simulink model "WSCC_Indian_400kV_Legacy"  (R2022a)
settings: Solver=FixedStepDiscrete  StartTime=0.0  StopTime=1  FixedStep=5e-7  RelTol=1e-3
PreLoadFcn:
  | tf=1e-3
  | to=20e-3
model workspace (MAT data in the model file):
  tf = 0.001
  to = 0.02
undefined symbols (not defined in the file or in its folder): D1, Delta
libraries: spsFourierLib x72, spsPowerPositiveSequenceLib x24, spsThreePhaseVIMeasurementLib x21, spsThreePhaseBreakerLib x12, spsDistributedParametersLineLib x12, spsLoadFlowBusLib x9, spsRMSLib x6, spsThreePhaseParallelRLCLoadLib x6, spsThreePhaseSeriesRLCLoadLib x3, spsThreePhaseSourceLib x3, spsThreePhaseTransformerTwoWindingsLib x3, spsThreePhaseFaultLib x1
(part 2 of 2)

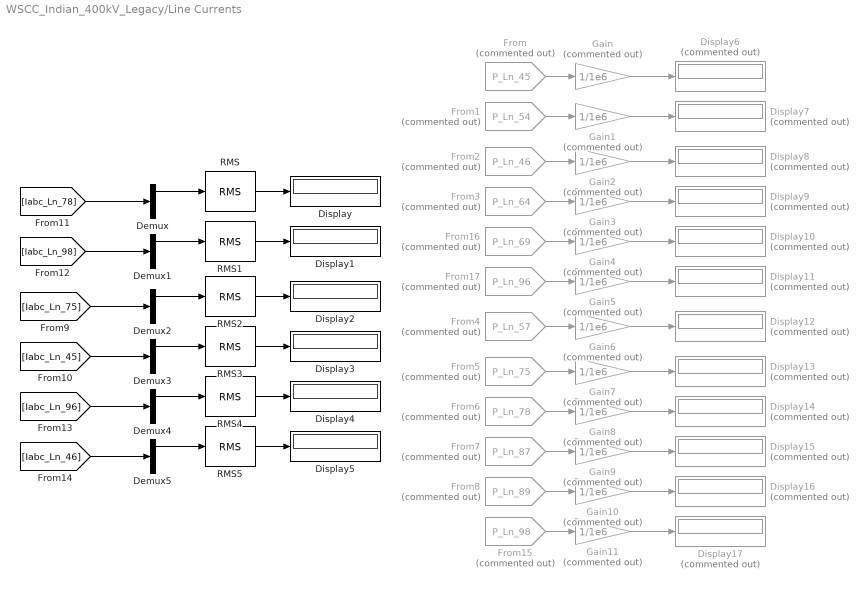
== system WSCC_Indian_400kV_Legacy/Line Currents ==
  Demux{,1..5} (6 alike) : Demux  Outputs=3
  Display{,1..5} (6 alike) : Display
  Display{6..17} (12 alike) : Display  Commented=on
  From : From  Commented=on  GotoTag=P_Ln_45  TagVisibility=global
  From1 : From  Commented=on  GotoTag=P_Ln_54  TagVisibility=global
  From15 : From  Commented=on  GotoTag=P_Ln_98  TagVisibility=global
  From16 : From  Commented=on  GotoTag=P_Ln_69  TagVisibility=global
  From17 : From  Commented=on  GotoTag=P_Ln_96  TagVisibility=global
  From2 : From  Commented=on  GotoTag=P_Ln_46  TagVisibility=global
  From3 : From  Commented=on  GotoTag=P_Ln_64  TagVisibility=global
  From4 : From  Commented=on  GotoTag=P_Ln_57  TagVisibility=global
  From5 : From  Commented=on  GotoTag=P_Ln_75  TagVisibility=global
  From6 : From  Commented=on  GotoTag=P_Ln_78  TagVisibility=global
  From7 : From  Commented=on  GotoTag=P_Ln_87  TagVisibility=global
  From8 : From  Commented=on  GotoTag=P_Ln_89  TagVisibility=global
  Gain{,1..11} (12 alike) : Gain  Commented=on  Gain=1/1e6
  RMS{,1..5} (6 alike) : spsRMSLib/RMS  TrueRMS=off  Freq=50  RMSInit=120  Ts=0
  wires:
  [Iabc_Ln_96] -> Demux4/1
  RMS4/1 -> Display4/1
  Demux5/1 -> RMS5/1
  Demux2/1 -> RMS2/1
  [Iabc_Ln_78] -> Demux/1
  Demux4/1 -> RMS4/1
  Demux3/1 -> RMS3/1
  RMS2/1 -> Display2/1
  RMS3/1 -> Display3/1
  Demux1/1 -> RMS1/1
  RMS1/1 -> Display1/1
  Demux/1 -> RMS/1
  [Iabc_Ln_46] -> Demux5/1
  [Iabc_Ln_45] -> Demux3/1
  [Iabc_Ln_75] -> Demux2/1
  [Iabc_Ln_98] -> Demux1/1
  RMS/1 -> Display/1
  RMS5/1 -> Display5/1
  From/1 -> Gain/1
  From1/1 -> Gain1/1
  From2/1 -> Gain2/1
  From3/1 -> Gain3/1
  From16/1 -> Gain4/1
  From17/1 -> Gain5/1
  From4/1 -> Gain6/1
  From5/1 -> Gain7/1
  From6/1 -> Gain8/1
  From7/1 -> Gain9/1
  From8/1 -> Gain10/1
  From15/1 -> Gain11/1
  Gain/1 -> Display6/1
  Gain1/1 -> Display7/1
  Gain2/1 -> Display8/1
  Gain3/1 -> Display9/1
  Gain4/1 -> Display10/1
  Gain5/1 -> Display11/1
  Gain6/1 -> Display12/1
  Gain7/1 -> Display13/1
  Gain8/1 -> Display14/1
  Gain9/1 -> Display15/1
  Gain10/1 -> Display16/1
  Gain11/1 -> Display17/1

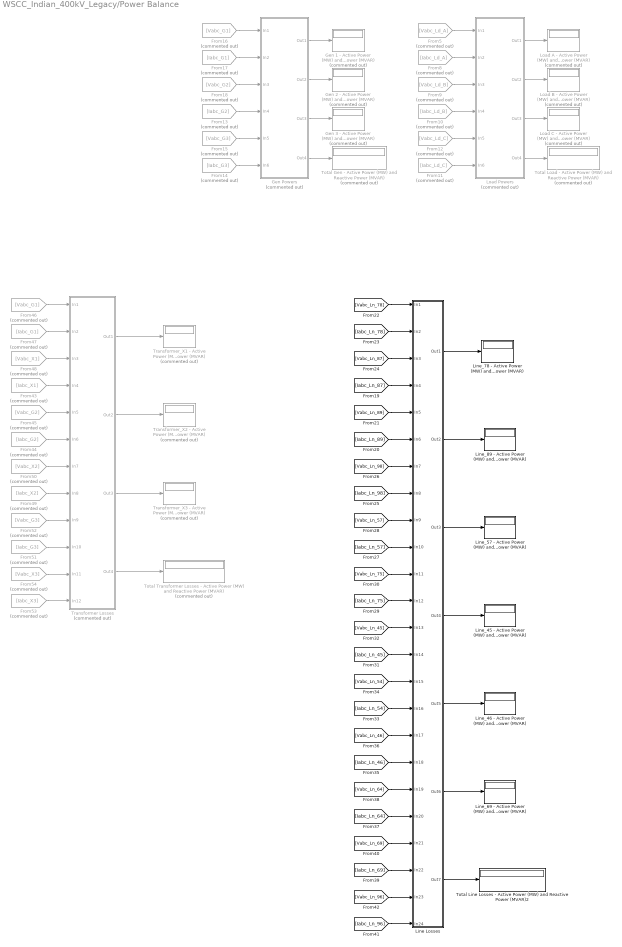
== system WSCC_Indian_400kV_Legacy/Power Balance ==
  From10 : From  Commented=on  GotoTag=Iabc_Ld_B  TagVisibility=global
  From11 : From  Commented=on  GotoTag=Iabc_Ld_C  TagVisibility=global
  From12 : From  Commented=on  GotoTag=Vabc_Ld_C  TagVisibility=global
  From13 : From  Commented=on  GotoTag=Iabc_G2  TagVisibility=global
  From14 : From  Commented=on  GotoTag=Iabc_G3  TagVisibility=global
  From15 : From  Commented=on  GotoTag=Vabc_G3  TagVisibility=global
  From16 : From  Commented=on  GotoTag=Vabc_G1  TagVisibility=global
  From17 : From  Commented=on  GotoTag=Iabc_G1  TagVisibility=global
  From18 : From  Commented=on  GotoTag=Vabc_G2  TagVisibility=global
  From43 : From  Commented=on  GotoTag=Iabc_X1  TagVisibility=global
  From44 : From  Commented=on  GotoTag=Iabc_G2  TagVisibility=global
  From45 : From  Commented=on  GotoTag=Vabc_G2  TagVisibility=global
  From46 : From  Commented=on  GotoTag=Vabc_G1  TagVisibility=global
  From47 : From  Commented=on  GotoTag=Iabc_G1  TagVisibility=global
  From48 : From  Commented=on  GotoTag=Vabc_X1  TagVisibility=global
  From49 : From  Commented=on  GotoTag=Iabc_X2  TagVisibility=global
  From5 : From  Commented=on  GotoTag=Vabc_Ld_A  TagVisibility=global
  From50 : From  Commented=on  GotoTag=Vabc_X2  TagVisibility=global
  From51 : From  Commented=on  GotoTag=Iabc_G3  TagVisibility=global
  From52 : From  Commented=on  GotoTag=Vabc_G3  TagVisibility=global
  From53 : From  Commented=on  GotoTag=Iabc_X3  TagVisibility=global
  From54 : From  Commented=on  GotoTag=Vabc_X3  TagVisibility=global
  From8 : From  Commented=on  GotoTag=Iabc_Ld_A  TagVisibility=global
  From9 : From  Commented=on  GotoTag=Vabc_Ld_B  TagVisibility=global
  Gen 1 - Active Power (MW) and Reactive Power (MVAR) : Display  Commented=on
  Gen 2 - Active Power (MW) and Reactive Power (MVAR) : Display  Commented=on
  Gen 3 - Active Power (MW) and Reactive Power (MVAR) : Display  Commented=on
  Gen Powers : Subsystem  Commented=on
  Line Losses : Subsystem
  Line_45 - Active Power (MW) and Reactive Power (MVAR) : Display
  Line_46 - Active Power (MW) and Reactive Power (MVAR) : Display
  Line_57 - Active Power (MW) and Reactive Power (MVAR) : Display
  Line_69 - Active Power (MW) and Reactive Power (MVAR) : Display
  Line_78 - Active Power (MW) and Reactive Power (MVAR) : Display
  Line_89 - Active Power (MW) and Reactive Power (MVAR) : Display
  Load A - Active Power (MW) and Reactive Power (MVAR) : Display  Commented=on
  Load B - Active Power (MW) and Reactive Power (MVAR) : Display  Commented=on
  Load C - Active Power (MW) and Reactive Power (MVAR) : Display  Commented=on
  Load Powers : Subsystem  Commented=on
  Total Gen - Active Power (MW) and Reactive Power (MVAR) : Display  Commented=on
  Total Line Losses - Active Power (MW) and Reactive Power (MVAR)2 : Display
  Total Load - Active Power (MW) and Reactive Power (MVAR) : Display  Commented=on
  Total Transformer Losses - Active Power (MW) and Reactive Power (MVAR) : Display  Commented=on
  Transformer Losses : Subsystem  Commented=on
  Transformer_X1 - Active Power (MW) and Reactive Power (MVAR) : Display  Commented=on
  Transformer_X2 - Active Power (MW) and Reactive Power (MVAR) : Display  Commented=on
  Transformer_X3 - Active Power (MW) and Reactive Power (MVAR) : Display  Commented=on
  wires:
  From44/1 -> Transformer Losses/6(In6)
  [Iabc_Ln_45] -> Line Losses/14(In14)
  From16/1 -> Gen Powers/1(In1)
  [Iabc_Ln_75] -> Line Losses/12(In12)
  Transformer Losses/1(Out1) -> Transformer_X1 - Active Power (MW) and Reactive Power (MVAR)/1
  Transformer Losses/4(Out4) -> Total Transformer Losses - Active Power (MW) and Reactive Power (MVAR)/1
  [Iabc_Ln_54] -> Line Losses/16(In16)
  [Vabc_Ln_54] -> Line Losses/15(In15)
  [Vabc_Ln_87] -> Line Losses/3(In3)
  From10/1 -> Load Powers/4(In4)
  [Vabc_Ln_98] -> Line Losses/7(In7)
  From11/1 -> Load Powers/6(In6)
  Line Losses/4(Out4) -> Line_45 - Active Power (MW) and Reactive Power (MVAR)/1
  Load Powers/4(Out4) -> Total Load - Active Power (MW) and Reactive Power (MVAR)/1
  Load Powers/3(Out3) -> Load C - Active Power (MW) and Reactive Power (MVAR)/1
  [Vabc_Ln_64] -> Line Losses/19(In19)
  From50/1 -> Transformer Losses/7(In7)
  Transformer Losses/2(Out2) -> Transformer_X2 - Active Power (MW) and Reactive Power (MVAR)/1
  [Vabc_Ln_57] -> Line Losses/9(In9)
  Line Losses/7(Out7) -> Total Line Losses - Active Power (MW) and Reactive Power (MVAR)2/1
  From48/1 -> Transformer Losses/3(In3)
  Load Powers/1(Out1) -> Load A - Active Power (MW) and Reactive Power (MVAR)/1
  From9/1 -> Load Powers/3(In3)
  [Iabc_Ln_46] -> Line Losses/18(In18)
  [Iabc_Ln_57] -> Line Losses/10(In10)
  [Iabc_Ln_69] -> Line Losses/22(In22)
  From52/1 -> Transformer Losses/9(In9)
  [Iabc_Ln_89] -> Line Losses/6(In6)
  Line Losses/2(Out2) -> Line_89 - Active Power (MW) and Reactive Power (MVAR)/1
  [Iabc_Ln_87] -> Line Losses/4(In4)
  From15/1 -> Gen Powers/5(In5)
  From18/1 -> Gen Powers/3(In3)
  [Vabc_Ln_69] -> Line Losses/21(In21)
  From51/1 -> Transformer Losses/10(In10)
  Transformer Losses/3(Out3) -> Transformer_X3 - Active Power (MW) and Reactive Power (MVAR)/1
  [Vabc_Ln_46] -> Line Losses/17(In17)
  Gen Powers/4(Out4) -> Total Gen - Active Power (MW) and Reactive Power (MVAR)/1
  [Iabc_Ln_98] -> Line Losses/8(In8)
  [Vabc_Ln_78] -> Line Losses/1(In1)
  From47/1 -> Transformer Losses/2(In2)
  From13/1 -> Gen Powers/4(In4)
  From53/1 -> Transformer Losses/12(In12)
  [Vabc_Ln_45] -> Line Losses/13(In13)
  From54/1 -> Transformer Losses/11(In11)
  [Iabc_Ln_96] -> Line Losses/24(In24)
  [Vabc_Ln_96] -> Line Losses/23(In23)
  From49/1 -> Transformer Losses/8(In8)
  [Vabc_Ln_75] -> Line Losses/11(In11)
  Gen Powers/1(Out1) -> Gen 1 - Active Power (MW) and Reactive Power (MVAR)/1
  [Vabc_Ln_89] -> Line Losses/5(In5)
  From8/1 -> Load Powers/2(In2)
  [Iabc_Ln_64] -> Line Losses/20(In20)
  From46/1 -> Transformer Losses/1(In1)
  From17/1 -> Gen Powers/2(In2)
  Line Losses/1(Out1) -> Line_78 - Active Power (MW) and Reactive Power (MVAR)/1
  Line Losses/3(Out3) -> Line_57 - Active Power (MW) and Reactive Power (MVAR)/1
  From45/1 -> Transformer Losses/5(In5)
  Line Losses/6(Out6) -> Line_69 - Active Power (MW) and Reactive Power (MVAR)/1
  [Iabc_Ln_78] -> Line Losses/2(In2)
  From14/1 -> Gen Powers/6(In6)
  Line Losses/5(Out5) -> Line_46 - Active Power (MW) and Reactive Power (MVAR)/1
  From43/1 -> Transformer Losses/4(In4)
  Gen Powers/3(Out3) -> Gen 3 - Active Power (MW) and Reactive Power (MVAR)/1
  Gen Powers/2(Out2) -> Gen 2 - Active Power (MW) and Reactive Power (MVAR)/1
  From5/1 -> Load Powers/1(In1)
  From12/1 -> Load Powers/5(In5)
  Load Powers/2(Out2) -> Load B - Active Power (MW) and Reactive Power (MVAR)/1

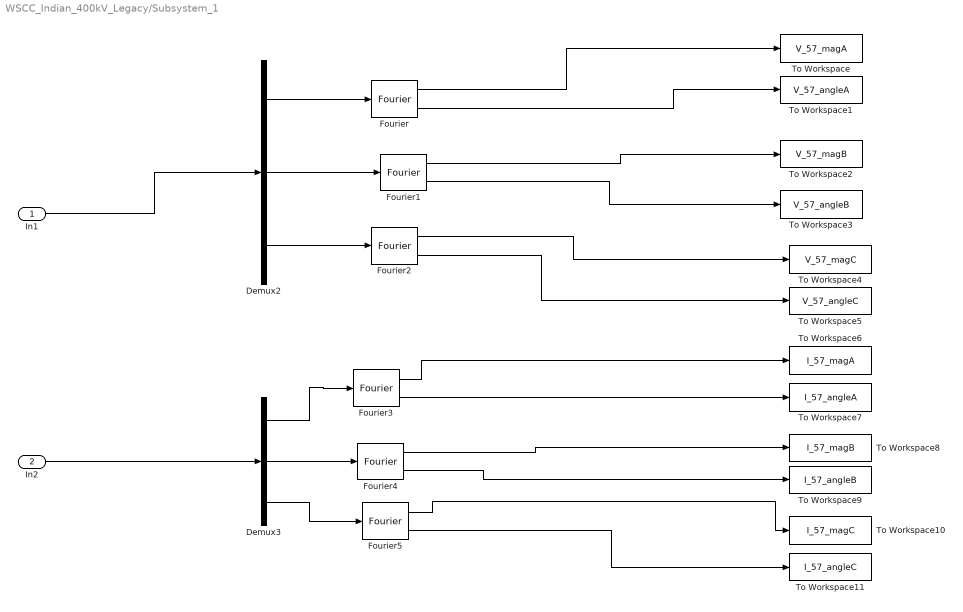
== system WSCC_Indian_400kV_Legacy/Subsystem_1 ==
  In1 : Inport
  In2 : Inport  Port=2
  Demux2 : Demux  Outputs=3
  Demux3 : Demux  Outputs=3
  Fourier{,1..5} (6 alike) : spsFourierLib/Fourier  Freq=50  n=1  InInit=[0, 0]  Ts=tf
      settings: SourceProductBaseCode=PS
  To Workspace : ToWorkspace  VariableName=V_57_magA  SaveFormat=Timeseries  SampleTime=to
  To Workspace1 : ToWorkspace  VariableName=V_57_angleA  SaveFormat=Timeseries  SampleTime=to
  To Workspace10 : ToWorkspace  VariableName=I_57_magC  SaveFormat=Timeseries  SampleTime=to
  To Workspace11 : ToWorkspace  VariableName=I_57_angleC  SaveFormat=Timeseries  SampleTime=to
  To Workspace2 : ToWorkspace  VariableName=V_57_magB  SaveFormat=Timeseries  SampleTime=to
  To Workspace3 : ToWorkspace  VariableName=V_57_angleB  SaveFormat=Timeseries  SampleTime=to
  To Workspace4 : ToWorkspace  VariableName=V_57_magC  SaveFormat=Timeseries  SampleTime=to
  To Workspace5 : ToWorkspace  VariableName=V_57_angleC  SaveFormat=Timeseries  SampleTime=to
  To Workspace6 : ToWorkspace  VariableName=I_57_magA  SaveFormat=Timeseries  SampleTime=to
  To Workspace7 : ToWorkspace  VariableName=I_57_angleA  SaveFormat=Timeseries  SampleTime=to
  To Workspace8 : ToWorkspace  VariableName=I_57_magB  SaveFormat=Timeseries  SampleTime=to
  To Workspace9 : ToWorkspace  VariableName=I_57_angleB  SaveFormat=Timeseries  SampleTime=to
  wires:
  Demux3/3 -> Fourier5/1
  Fourier4/1 -> To Workspace8/1
  Demux3/2 -> Fourier4/1
  Fourier3/2 -> To Workspace7/1
  Fourier5/1 -> To Workspace10/1
  Fourier3/1 -> To Workspace6/1
  Fourier5/2 -> To Workspace11/1
  Fourier4/2 -> To Workspace9/1
  Fourier2/2 -> To Workspace5/1
  Demux3/1 -> Fourier3/1
  Fourier2/1 -> To Workspace4/1
  Fourier1/2 -> To Workspace3/1
  Demux2/2 -> Fourier1/1
  Fourier/2 -> To Workspace1/1
  Fourier1/1 -> To Workspace2/1
  Demux2/3 -> Fourier2/1
  Fourier/1 -> To Workspace/1
  Demux2/1 -> Fourier/1
  In1/1 -> Demux2/1
  In2/1 -> Demux3/1

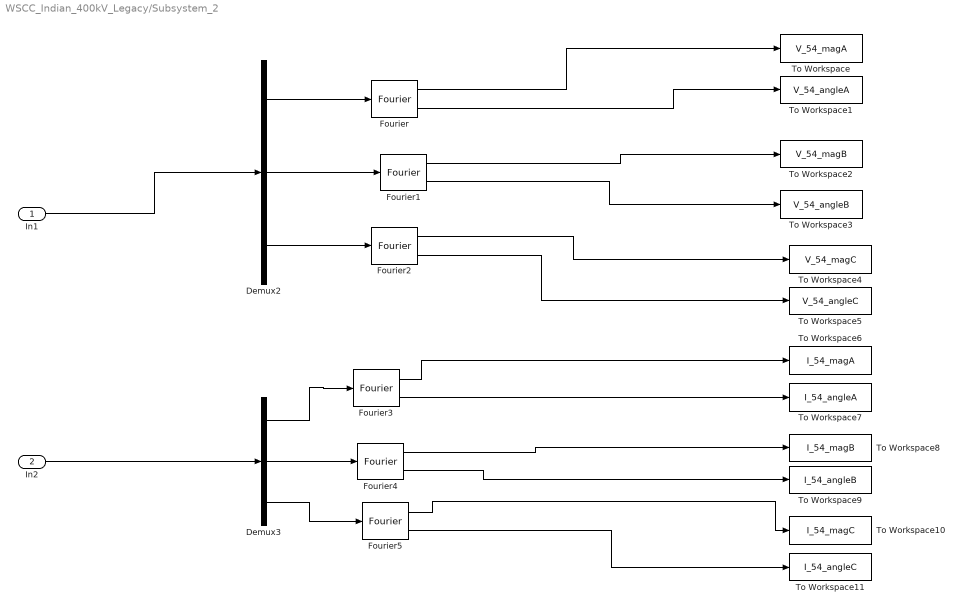
== system WSCC_Indian_400kV_Legacy/Subsystem_2 ==
  In1 : Inport
  In2 : Inport  Port=2
  Demux2 : Demux  Outputs=3
  Demux3 : Demux  Outputs=3
  Fourier{,1..5} (6 alike) : spsFourierLib/Fourier  Freq=50  n=1  InInit=[0, 0]  Ts=tf
      settings: SourceProductBaseCode=PS
  To Workspace : ToWorkspace  VariableName=V_54_magA  SaveFormat=Timeseries  SampleTime=to
  To Workspace1 : ToWorkspace  VariableName=V_54_angleA  SaveFormat=Timeseries  SampleTime=to
  To Workspace10 : ToWorkspace  VariableName=I_54_magC  SaveFormat=Timeseries  SampleTime=to
  To Workspace11 : ToWorkspace  VariableName=I_54_angleC  SaveFormat=Timeseries  SampleTime=to
  To Workspace2 : ToWorkspace  VariableName=V_54_magB  SaveFormat=Timeseries  SampleTime=to
  To Workspace3 : ToWorkspace  VariableName=V_54_angleB  SaveFormat=Timeseries  SampleTime=to
  To Workspace4 : ToWorkspace  VariableName=V_54_magC  SaveFormat=Timeseries  SampleTime=to
  To Workspace5 : ToWorkspace  VariableName=V_54_angleC  SaveFormat=Timeseries  SampleTime=to
  To Workspace6 : ToWorkspace  VariableName=I_54_magA  SaveFormat=Timeseries  SampleTime=to
  To Workspace7 : ToWorkspace  VariableName=I_54_angleA  SaveFormat=Timeseries  SampleTime=to
  To Workspace8 : ToWorkspace  VariableName=I_54_magB  SaveFormat=Timeseries  SampleTime=to
  To Workspace9 : ToWorkspace  VariableName=I_54_angleB  SaveFormat=Timeseries  SampleTime=to
  wires:
  Demux3/3 -> Fourier5/1
  Fourier4/1 -> To Workspace8/1
  Demux3/2 -> Fourier4/1
  Fourier3/2 -> To Workspace7/1
  Fourier5/1 -> To Workspace10/1
  Fourier3/1 -> To Workspace6/1
  Fourier5/2 -> To Workspace11/1
  Fourier4/2 -> To Workspace9/1
  Fourier2/2 -> To Workspace5/1
  Demux3/1 -> Fourier3/1
  Fourier2/1 -> To Workspace4/1
  Fourier1/2 -> To Workspace3/1
  Demux2/2 -> Fourier1/1
  Fourier/2 -> To Workspace1/1
  Fourier1/1 -> To Workspace2/1
  Demux2/3 -> Fourier2/1
  Fourier/1 -> To Workspace/1
  Demux2/1 -> Fourier/1
  In1/1 -> Demux2/1
  In2/1 -> Demux3/1

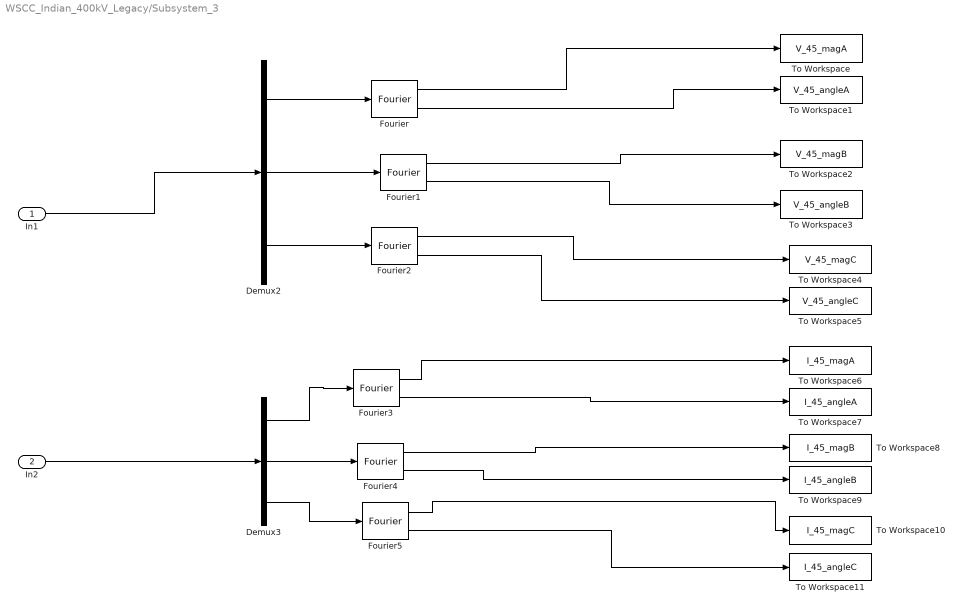
== system WSCC_Indian_400kV_Legacy/Subsystem_3 ==
  In1 : Inport
  In2 : Inport  Port=2
  Demux2 : Demux  Outputs=3
  Demux3 : Demux  Outputs=3
  Fourier{,1..5} (6 alike) : spsFourierLib/Fourier  Freq=50  n=1  InInit=[0, 0]  Ts=tf
      settings: SourceProductBaseCode=PS
  To Workspace : ToWorkspace  VariableName=V_45_magA  SaveFormat=Timeseries  SampleTime=to
  To Workspace1 : ToWorkspace  VariableName=V_45_angleA  SaveFormat=Timeseries  SampleTime=to
  To Workspace10 : ToWorkspace  VariableName=I_45_magC  SaveFormat=Timeseries  SampleTime=to
  To Workspace11 : ToWorkspace  VariableName=I_45_angleC  SaveFormat=Timeseries  SampleTime=to
  To Workspace2 : ToWorkspace  VariableName=V_45_magB  SaveFormat=Timeseries  SampleTime=to
  To Workspace3 : ToWorkspace  VariableName=V_45_angleB  SaveFormat=Timeseries  SampleTime=to
  To Workspace4 : ToWorkspace  VariableName=V_45_magC  SaveFormat=Timeseries  SampleTime=to
  To Workspace5 : ToWorkspace  VariableName=V_45_angleC  SaveFormat=Timeseries  SampleTime=to
  To Workspace6 : ToWorkspace  VariableName=I_45_magA  SaveFormat=Timeseries  SampleTime=to
  To Workspace7 : ToWorkspace  VariableName=I_45_angleA  SaveFormat=Timeseries  SampleTime=to
  To Workspace8 : ToWorkspace  VariableName=I_45_magB  SaveFormat=Timeseries  SampleTime=to
  To Workspace9 : ToWorkspace  VariableName=I_45_angleB  SaveFormat=Timeseries  SampleTime=to
  wires:
  Demux3/3 -> Fourier5/1
  Fourier4/1 -> To Workspace8/1
  Demux3/2 -> Fourier4/1
  Fourier3/2 -> To Workspace7/1
  Fourier5/1 -> To Workspace10/1
  Fourier3/1 -> To Workspace6/1
  Fourier5/2 -> To Workspace11/1
  Fourier4/2 -> To Workspace9/1
  Fourier2/2 -> To Workspace5/1
  Demux3/1 -> Fourier3/1
  Fourier2/1 -> To Workspace4/1
  Fourier1/2 -> To Workspace3/1
  Demux2/2 -> Fourier1/1
  Fourier/2 -> To Workspace1/1
  Fourier1/1 -> To Workspace2/1
  Demux2/3 -> Fourier2/1
  Fourier/1 -> To Workspace/1
  Demux2/1 -> Fourier/1
  In1/1 -> Demux2/1
  In2/1 -> Demux3/1

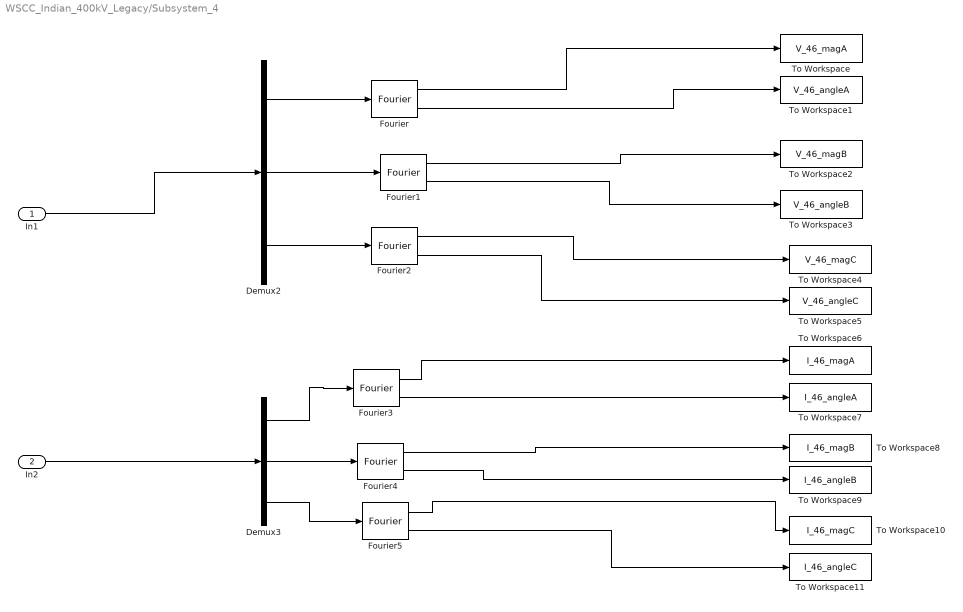
== system WSCC_Indian_400kV_Legacy/Subsystem_4 ==
  In1 : Inport
  In2 : Inport  Port=2
  Demux2 : Demux  Outputs=3
  Demux3 : Demux  Outputs=3
  Fourier{,1..5} (6 alike) : spsFourierLib/Fourier  Freq=50  n=1  InInit=[0, 0]  Ts=tf
      settings: SourceProductBaseCode=PS
  To Workspace : ToWorkspace  VariableName=V_46_magA  SaveFormat=Timeseries  SampleTime=to
  To Workspace1 : ToWorkspace  VariableName=V_46_angleA  SaveFormat=Timeseries  SampleTime=to
  To Workspace10 : ToWorkspace  VariableName=I_46_magC  SaveFormat=Timeseries  SampleTime=to
  To Workspace11 : ToWorkspace  VariableName=I_46_angleC  SaveFormat=Timeseries  SampleTime=to
  To Workspace2 : ToWorkspace  VariableName=V_46_magB  SaveFormat=Timeseries  SampleTime=to
  To Workspace3 : ToWorkspace  VariableName=V_46_angleB  SaveFormat=Timeseries  SampleTime=to
  To Workspace4 : ToWorkspace  VariableName=V_46_magC  SaveFormat=Timeseries  SampleTime=to
  To Workspace5 : ToWorkspace  VariableName=V_46_angleC  SaveFormat=Timeseries  SampleTime=to
  To Workspace6 : ToWorkspace  VariableName=I_46_magA  SaveFormat=Timeseries  SampleTime=to
  To Workspace7 : ToWorkspace  VariableName=I_46_angleA  SaveFormat=Timeseries  SampleTime=to
  To Workspace8 : ToWorkspace  VariableName=I_46_magB  SaveFormat=Timeseries  SampleTime=to
  To Workspace9 : ToWorkspace  VariableName=I_46_angleB  SaveFormat=Timeseries  SampleTime=to
  wires:
  Demux3/3 -> Fourier5/1
  Fourier4/1 -> To Workspace8/1
  Demux3/2 -> Fourier4/1
  Fourier3/2 -> To Workspace7/1
  Fourier5/1 -> To Workspace10/1
  Fourier3/1 -> To Workspace6/1
  Fourier5/2 -> To Workspace11/1
  Fourier4/2 -> To Workspace9/1
  Fourier2/2 -> To Workspace5/1
  Demux3/1 -> Fourier3/1
  Fourier2/1 -> To Workspace4/1
  Fourier1/2 -> To Workspace3/1
  Demux2/2 -> Fourier1/1
  Fourier/2 -> To Workspace1/1
  Fourier1/1 -> To Workspace2/1
  Demux2/3 -> Fourier2/1
  Fourier/1 -> To Workspace/1
  Demux2/1 -> Fourier/1
  In1/1 -> Demux2/1
  In2/1 -> Demux3/1

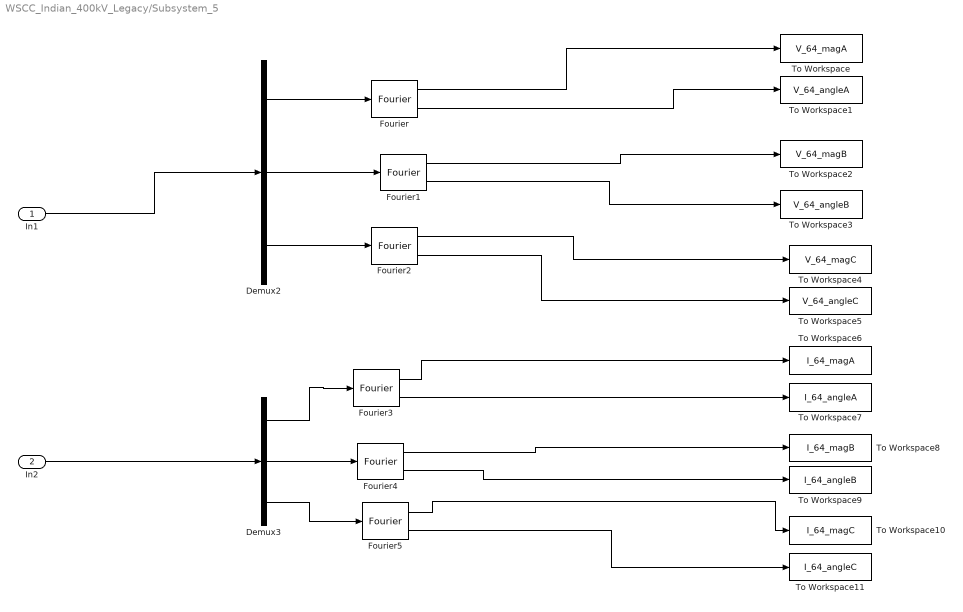
== system WSCC_Indian_400kV_Legacy/Subsystem_5 ==
  In1 : Inport
  In2 : Inport  Port=2
  Demux2 : Demux  Outputs=3
  Demux3 : Demux  Outputs=3
  Fourier{,1..5} (6 alike) : spsFourierLib/Fourier  Freq=50  n=1  InInit=[0, 0]  Ts=tf
      settings: SourceProductBaseCode=PS
  To Workspace : ToWorkspace  VariableName=V_64_magA  SaveFormat=Timeseries  SampleTime=to
  To Workspace1 : ToWorkspace  VariableName=V_64_angleA  SaveFormat=Timeseries  SampleTime=to
  To Workspace10 : ToWorkspace  VariableName=I_64_magC  SaveFormat=Timeseries  SampleTime=to
  To Workspace11 : ToWorkspace  VariableName=I_64_angleC  SaveFormat=Timeseries  SampleTime=to
  To Workspace2 : ToWorkspace  VariableName=V_64_magB  SaveFormat=Timeseries  SampleTime=to
  To Workspace3 : ToWorkspace  VariableName=V_64_angleB  SaveFormat=Timeseries  SampleTime=to
  To Workspace4 : ToWorkspace  VariableName=V_64_magC  SaveFormat=Timeseries  SampleTime=to
  To Workspace5 : ToWorkspace  VariableName=V_64_angleC  SaveFormat=Timeseries  SampleTime=to
  To Workspace6 : ToWorkspace  VariableName=I_64_magA  SaveFormat=Timeseries  SampleTime=to
  To Workspace7 : ToWorkspace  VariableName=I_64_angleA  SaveFormat=Timeseries  SampleTime=to
  To Workspace8 : ToWorkspace  VariableName=I_64_magB  SaveFormat=Timeseries  SampleTime=to
  To Workspace9 : ToWorkspace  VariableName=I_64_angleB  SaveFormat=Timeseries  SampleTime=to
  wires:
  Demux3/3 -> Fourier5/1
  Fourier4/1 -> To Workspace8/1
  Demux3/2 -> Fourier4/1
  Fourier3/2 -> To Workspace7/1
  Fourier5/1 -> To Workspace10/1
  Fourier3/1 -> To Workspace6/1
  Fourier5/2 -> To Workspace11/1
  Fourier4/2 -> To Workspace9/1
  Fourier2/2 -> To Workspace5/1
  Demux3/1 -> Fourier3/1
  Fourier2/1 -> To Workspace4/1
  Fourier1/2 -> To Workspace3/1
  Demux2/2 -> Fourier1/1
  Fourier/2 -> To Workspace1/1
  Fourier1/1 -> To Workspace2/1
  Demux2/3 -> Fourier2/1
  Fourier/1 -> To Workspace/1
  Demux2/1 -> Fourier/1
  In1/1 -> Demux2/1
  In2/1 -> Demux3/1

== system WSCC_Indian_400kV_Legacy/Subsystem_6 ==
  In1 : Inport
  In2 : Inport  Port=2
  Demux2 : Demux  Outputs=3
  Demux3 : Demux  Outputs=3
  Fourier{,1..5} (6 alike) : spsFourierLib/Fourier  Freq=50  n=1  InInit=[0, 0]  Ts=tf
      settings: SourceProductBaseCode=PS
  To Workspace : ToWorkspace  VariableName=V_69_magA  SaveFormat=Timeseries  SampleTime=to
  To Workspace1 : ToWorkspace  VariableName=V_69_angleA  SaveFormat=Timeseries  SampleTime=to
  To Workspace10 : ToWorkspace  VariableName=I_69_magC  SaveFormat=Timeseries  SampleTime=to
  To Workspace11 : ToWorkspace  VariableName=I_69_angleC  SaveFormat=Timeseries  SampleTime=to
  To Workspace2 : ToWorkspace  VariableName=V_69_magB  SaveFormat=Timeseries  SampleTime=to
  To Workspace3 : ToWorkspace  VariableName=V_69_angleB  SaveFormat=Timeseries  SampleTime=to
  To Workspace4 : ToWorkspace  VariableName=V_69_magC  SaveFormat=Timeseries  SampleTime=to
  To Workspace5 : ToWorkspace  VariableName=V_69_angleC  SaveFormat=Timeseries  SampleTime=to
  To Workspace6 : ToWorkspace  VariableName=I_69_magA  SaveFormat=Timeseries  SampleTime=to
  To Workspace7 : ToWorkspace  VariableName=I_69_angleA  SaveFormat=Timeseries  SampleTime=to
  To Workspace8 : ToWorkspace  VariableName=I_69_magB  SaveFormat=Timeseries  SampleTime=to
  To Workspace9 : ToWorkspace  VariableName=I_69_angleB  SaveFormat=Timeseries  SampleTime=to
  wires:
  Demux3/3 -> Fourier5/1
  Fourier4/1 -> To Workspace8/1
  Demux3/2 -> Fourier4/1
  Fourier3/2 -> To Workspace7/1
  Fourier5/1 -> To Workspace10/1
  Fourier3/1 -> To Workspace6/1
  Fourier5/2 -> To Workspace11/1
  Fourier4/2 -> To Workspace9/1
  Fourier2/2 -> To Workspace5/1
  Demux3/1 -> Fourier3/1
  Fourier2/1 -> To Workspace4/1
  Fourier1/2 -> To Workspace3/1
  Demux2/2 -> Fourier1/1
  Fourier/2 -> To Workspace1/1
  Fourier1/1 -> To Workspace2/1
  Demux2/3 -> Fourier2/1
  Fourier/1 -> To Workspace/1
  Demux2/1 -> Fourier/1
  In1/1 -> Demux2/1
  In2/1 -> Demux3/1

== system WSCC_Indian_400kV_Legacy/Subsystem_7 ==
  In1 : Inport
  In2 : Inport  Port=2
  Demux2 : Demux  Outputs=3
  Demux3 : Demux  Outputs=3
  Fourier{,1..5} (6 alike) : spsFourierLib/Fourier  Freq=50  n=1  InInit=[0, 0]  Ts=tf
      settings: SourceProductBaseCode=PS
  To Workspace : ToWorkspace  VariableName=V_96_magA  SaveFormat=Timeseries  SampleTime=to
  To Workspace1 : ToWorkspace  VariableName=V_96_angleA  SaveFormat=Timeseries  SampleTime=to
  To Workspace10 : ToWorkspace  VariableName=I_96_magC  SaveFormat=Timeseries  SampleTime=to
  To Workspace11 : ToWorkspace  VariableName=I_96_angleC  SaveFormat=Timeseries  SampleTime=to
  To Workspace2 : ToWorkspace  VariableName=V_96_magB  SaveFormat=Timeseries  SampleTime=to
  To Workspace3 : ToWorkspace  VariableName=V_96_angleB  SaveFormat=Timeseries  SampleTime=to
  To Workspace4 : ToWorkspace  VariableName=V_96_magC  SaveFormat=Timeseries  SampleTime=to
  To Workspace5 : ToWorkspace  VariableName=V_96_angleC  SaveFormat=Timeseries  SampleTime=to
  To Workspace6 : ToWorkspace  VariableName=I_96_magA  SaveFormat=Timeseries  SampleTime=to
  To Workspace7 : ToWorkspace  VariableName=I_96_angleA  SaveFormat=Timeseries  SampleTime=to
  To Workspace8 : ToWorkspace  VariableName=I_96_magB  SaveFormat=Timeseries  SampleTime=to
  To Workspace9 : ToWorkspace  VariableName=I_96_angleB  SaveFormat=Timeseries  SampleTime=to
  wires:
  Demux3/3 -> Fourier5/1
  Fourier4/1 -> To Workspace8/1
  Demux3/2 -> Fourier4/1
  Fourier3/2 -> To Workspace7/1
  Fourier5/1 -> To Workspace10/1
  Fourier3/1 -> To Workspace6/1
  Fourier5/2 -> To Workspace11/1
  Fourier4/2 -> To Workspace9/1
  Fourier2/2 -> To Workspace5/1
  Demux3/1 -> Fourier3/1
  Fourier2/1 -> To Workspace4/1
  Fourier1/2 -> To Workspace3/1
  Demux2/2 -> Fourier1/1
  Fourier/2 -> To Workspace1/1
  Fourier1/1 -> To Workspace2/1
  Demux2/3 -> Fourier2/1
  Fourier/1 -> To Workspace/1
  Demux2/1 -> Fourier/1
  In1/1 -> Demux2/1
  In2/1 -> Demux3/1

== system WSCC_Indian_400kV_Legacy/Subsystem_75 ==
  In1 : Inport
  In2 : Inport  Port=2
  Demux2 : Demux  Outputs=3
  Demux3 : Demux  Outputs=3
  Fourier{,1..5} (6 alike) : spsFourierLib/Fourier  Freq=50  n=1  InInit=[0, 0]  Ts=tf
      settings: SourceProductBaseCode=PS
  To Workspace : ToWorkspace  VariableName=V_75_magA  SaveFormat=Timeseries  SampleTime=to
  To Workspace1 : ToWorkspace  VariableName=V_75_angleA  SaveFormat=Timeseries  SampleTime=to
  To Workspace10 : ToWorkspace  VariableName=I_75_magC  SaveFormat=Timeseries  SampleTime=to
  To Workspace11 : ToWorkspace  VariableName=I_75_angleC  SaveFormat=Timeseries  SampleTime=to
  To Workspace2 : ToWorkspace  VariableName=V_75_magB  SaveFormat=Timeseries  SampleTime=to
  To Workspace3 : ToWorkspace  VariableName=V_75_angleB  SaveFormat=Timeseries  SampleTime=to
  To Workspace4 : ToWorkspace  VariableName=V_75_magC  SaveFormat=Timeseries  SampleTime=to
  To Workspace5 : ToWorkspace  VariableName=V_75_angleC  SaveFormat=Timeseries  SampleTime=to
  To Workspace6 : ToWorkspace  VariableName=I_75_magA  SaveFormat=Timeseries  SampleTime=to
  To Workspace7 : ToWorkspace  VariableName=I_75_angleA  SaveFormat=Timeseries  SampleTime=to
  To Workspace8 : ToWorkspace  VariableName=I_75_magB  SaveFormat=Timeseries  SampleTime=to
  To Workspace9 : ToWorkspace  VariableName=I_75_angleB  SaveFormat=Timeseries  SampleTime=to
  wires:
  Demux3/3 -> Fourier5/1
  Fourier4/1 -> To Workspace8/1
  Demux3/2 -> Fourier4/1
  Fourier3/2 -> To Workspace7/1
  Fourier5/1 -> To Workspace10/1
  Fourier3/1 -> To Workspace6/1
  Fourier5/2 -> To Workspace11/1
  Fourier4/2 -> To Workspace9/1
  Fourier2/2 -> To Workspace5/1
  Demux3/1 -> Fourier3/1
  Fourier2/1 -> To Workspace4/1
  Fourier1/2 -> To Workspace3/1
  Demux2/2 -> Fourier1/1
  Fourier/2 -> To Workspace1/1
  Fourier1/1 -> To Workspace2/1
  Demux2/3 -> Fourier2/1
  Fourier/1 -> To Workspace/1
  Demux2/1 -> Fourier/1
  In1/1 -> Demux2/1
  In2/1 -> Demux3/1

== system WSCC_Indian_400kV_Legacy/Subsystem_78 ==
  In1 : Inport
  In2 : Inport  Port=2
  Demux2 : Demux  Outputs=3
  Demux3 : Demux  Outputs=3
  Fourier{,1..5} (6 alike) : spsFourierLib/Fourier  Freq=50  n=1  InInit=[0, 0]  Ts=tf
      settings: SourceProductBaseCode=PS
  To Workspace : ToWorkspace  VariableName=V_78_magA  SaveFormat=Timeseries  SampleTime=to
  To Workspace1 : ToWorkspace  VariableName=V_78_angleA  SaveFormat=Timeseries  SampleTime=to
  To Workspace10 : ToWorkspace  VariableName=I_78_magC  SaveFormat=Timeseries  SampleTime=to
  To Workspace11 : ToWorkspace  VariableName=I_78_angleC  SaveFormat=Timeseries  SampleTime=to
  To Workspace2 : ToWorkspace  VariableName=V_78_magB  SaveFormat=Timeseries  SampleTime=to
  To Workspace3 : ToWorkspace  VariableName=V_78_angleB  SaveFormat=Timeseries  SampleTime=to
  To Workspace4 : ToWorkspace  VariableName=V_78_magC  SaveFormat=Timeseries  SampleTime=to
  To Workspace5 : ToWorkspace  VariableName=V_78_angleC  SaveFormat=Timeseries  SampleTime=to
  To Workspace6 : ToWorkspace  VariableName=I_78_magA  SaveFormat=Timeseries  SampleTime=to
  To Workspace7 : ToWorkspace  VariableName=I_78_angleA  SaveFormat=Timeseries  SampleTime=to
  To Workspace8 : ToWorkspace  VariableName=I_78_magB  SaveFormat=Timeseries  SampleTime=to
  To Workspace9 : ToWorkspace  VariableName=I_78_angleB  SaveFormat=Timeseries  SampleTime=to
  wires:
  Demux3/3 -> Fourier5/1
  Fourier4/1 -> To Workspace8/1
  Demux3/2 -> Fourier4/1
  Fourier3/2 -> To Workspace7/1
  Fourier5/1 -> To Workspace10/1
  Fourier3/1 -> To Workspace6/1
  Fourier5/2 -> To Workspace11/1
  Fourier4/2 -> To Workspace9/1
  Fourier2/2 -> To Workspace5/1
  Demux3/1 -> Fourier3/1
  Fourier2/1 -> To Workspace4/1
  Fourier1/2 -> To Workspace3/1
  Demux2/2 -> Fourier1/1
  Fourier/2 -> To Workspace1/1
  Fourier1/1 -> To Workspace2/1
  Demux2/3 -> Fourier2/1
  Fourier/1 -> To Workspace/1
  Demux2/1 -> Fourier/1
  In1/1 -> Demux2/1
  In2/1 -> Demux3/1

== system WSCC_Indian_400kV_Legacy/Subsystem_8 ==
  In1 : Inport
  In2 : Inport  Port=2
  Demux2 : Demux  Outputs=3
  Demux3 : Demux  Outputs=3
  Fourier{,1..5} (6 alike) : spsFourierLib/Fourier  Freq=50  n=1  InInit=[0, 0]  Ts=tf
      settings: SourceProductBaseCode=PS
  To Workspace : ToWorkspace  VariableName=V_89_magA  SaveFormat=Timeseries  SampleTime=to
  To Workspace1 : ToWorkspace  VariableName=V_89_angleA  SaveFormat=Timeseries  SampleTime=to
  To Workspace10 : ToWorkspace  VariableName=I_89_magC  SaveFormat=Timeseries  SampleTime=to
  To Workspace11 : ToWorkspace  VariableName=I_89_angleC  SaveFormat=Timeseries  SampleTime=to
  To Workspace2 : ToWorkspace  VariableName=V_89_magB  SaveFormat=Timeseries  SampleTime=to
  To Workspace3 : ToWorkspace  VariableName=V_89_angleB  SaveFormat=Timeseries  SampleTime=to
  To Workspace4 : ToWorkspace  VariableName=V_89_magC  SaveFormat=Timeseries  SampleTime=to
  To Workspace5 : ToWorkspace  VariableName=V_89_angleC  SaveFormat=Timeseries  SampleTime=to
  To Workspace6 : ToWorkspace  VariableName=I_89_magA  SaveFormat=Timeseries  SampleTime=to
  To Workspace7 : ToWorkspace  VariableName=I_89_angleA  SaveFormat=Timeseries  SampleTime=to
  To Workspace8 : ToWorkspace  VariableName=I_89_magB  SaveFormat=Timeseries  SampleTime=to
  To Workspace9 : ToWorkspace  VariableName=I_89_angleB  SaveFormat=Timeseries  SampleTime=to
  wires:
  Demux3/3 -> Fourier5/1
  Fourier4/1 -> To Workspace8/1
  Demux3/2 -> Fourier4/1
  Fourier3/2 -> To Workspace7/1
  Fourier5/1 -> To Workspace10/1
  Fourier3/1 -> To Workspace6/1
  Fourier5/2 -> To Workspace11/1
  Fourier4/2 -> To Workspace9/1
  Fourier2/2 -> To Workspace5/1
  Demux3/1 -> Fourier3/1
  Fourier2/1 -> To Workspace4/1
  Fourier1/2 -> To Workspace3/1
  Demux2/2 -> Fourier1/1
  Fourier/2 -> To Workspace1/1
  Fourier1/1 -> To Workspace2/1
  Demux2/3 -> Fourier2/1
  Fourier/1 -> To Workspace/1
  Demux2/1 -> Fourier/1
  In1/1 -> Demux2/1
  In2/1 -> Demux3/1

== system WSCC_Indian_400kV_Legacy/Subsystem_87 ==
  In1 : Inport
  In2 : Inport  Port=2
  Demux2 : Demux  Outputs=3
  Demux3 : Demux  Outputs=3
  Fourier{,1..5} (6 alike) : spsFourierLib/Fourier  Freq=50  n=1  InInit=[0, 0]  Ts=tf
      settings: SourceProductBaseCode=PS
  To Workspace : ToWorkspace  VariableName=V_87_magA  SaveFormat=Timeseries  SampleTime=to
  To Workspace1 : ToWorkspace  VariableName=V_87_angleA  SaveFormat=Timeseries  SampleTime=to
  To Workspace10 : ToWorkspace  VariableName=I_87_magC  SaveFormat=Timeseries  SampleTime=to
  To Workspace11 : ToWorkspace  VariableName=I_87_angleC  SaveFormat=Timeseries  SampleTime=to
  To Workspace2 : ToWorkspace  VariableName=V_87_magB  SaveFormat=Timeseries  SampleTime=to
  To Workspace3 : ToWorkspace  VariableName=V_87_angleB  SaveFormat=Timeseries  SampleTime=to
  To Workspace4 : ToWorkspace  VariableName=V_87_magC  SaveFormat=Timeseries  SampleTime=to
  To Workspace5 : ToWorkspace  VariableName=V_87_angleC  SaveFormat=Timeseries  SampleTime=to
  To Workspace6 : ToWorkspace  VariableName=I_87_magA  SaveFormat=Timeseries  SampleTime=to
  To Workspace7 : ToWorkspace  VariableName=I_87_angleA  SaveFormat=Timeseries  SampleTime=to
  To Workspace8 : ToWorkspace  VariableName=I_87_magB  SaveFormat=Timeseries  SampleTime=to
  To Workspace9 : ToWorkspace  VariableName=I_87_angleB  SaveFormat=Timeseries  SampleTime=to
  wires:
  Demux3/3 -> Fourier5/1
  Fourier4/1 -> To Workspace8/1
  Demux3/2 -> Fourier4/1
  Fourier3/2 -> To Workspace7/1
  Fourier5/1 -> To Workspace10/1
  Fourier3/1 -> To Workspace6/1
  Fourier5/2 -> To Workspace11/1
  Fourier4/2 -> To Workspace9/1
  Fourier2/2 -> To Workspace5/1
  Demux3/1 -> Fourier3/1
  Fourier2/1 -> To Workspace4/1
  Fourier1/2 -> To Workspace3/1
  Demux2/2 -> Fourier1/1
  Fourier/2 -> To Workspace1/1
  Fourier1/1 -> To Workspace2/1
  Demux2/3 -> Fourier2/1
  Fourier/1 -> To Workspace/1
  Demux2/1 -> Fourier/1
  In1/1 -> Demux2/1
  In2/1 -> Demux3/1

== system WSCC_Indian_400kV_Legacy/Subsystem_9 ==
  In1 : Inport
  In2 : Inport  Port=2
  Demux2 : Demux  Outputs=3
  Demux3 : Demux  Outputs=3
  Fourier{,1..5} (6 alike) : spsFourierLib/Fourier  Freq=50  n=1  InInit=[0, 0]  Ts=tf
      settings: SourceProductBaseCode=PS
  To Workspace : ToWorkspace  VariableName=V_98_magA  SaveFormat=Timeseries  SampleTime=to
  To Workspace1 : ToWorkspace  VariableName=V_98_angleA  SaveFormat=Timeseries  SampleTime=to
  To Workspace10 : ToWorkspace  VariableName=I_98_magC  SaveFormat=Timeseries  SampleTime=to
  To Workspace11 : ToWorkspace  VariableName=I_98_angleC  SaveFormat=Timeseries  SampleTime=to
  To Workspace2 : ToWorkspace  VariableName=V_98_magB  SaveFormat=Timeseries  SampleTime=to
  To Workspace3 : ToWorkspace  VariableName=V_98_angleB  SaveFormat=Timeseries  SampleTime=to
  To Workspace4 : ToWorkspace  VariableName=V_98_magC  SaveFormat=Timeseries  SampleTime=to
  To Workspace5 : ToWorkspace  VariableName=V_98_angleC  SaveFormat=Timeseries  SampleTime=to
  To Workspace6 : ToWorkspace  VariableName=I_98_magA  SaveFormat=Timeseries  SampleTime=to
  To Workspace7 : ToWorkspace  VariableName=I_98_angleA  SaveFormat=Timeseries  SampleTime=to
  To Workspace8 : ToWorkspace  VariableName=I_98_magB  SaveFormat=Timeseries  SampleTime=to
  To Workspace9 : ToWorkspace  VariableName=I_98_angleB  SaveFormat=Timeseries  SampleTime=to
  wires:
  Demux3/3 -> Fourier5/1
  Fourier4/1 -> To Workspace8/1
  Demux3/2 -> Fourier4/1
  Fourier3/2 -> To Workspace7/1
  Fourier5/1 -> To Workspace10/1
  Fourier3/1 -> To Workspace6/1
  Fourier5/2 -> To Workspace11/1
  Fourier4/2 -> To Workspace9/1
  Fourier2/2 -> To Workspace5/1
  Demux3/1 -> Fourier3/1
  Fourier2/1 -> To Workspace4/1
  Fourier1/2 -> To Workspace3/1
  Demux2/2 -> Fourier1/1
  Fourier/2 -> To Workspace1/1
  Fourier1/1 -> To Workspace2/1
  Demux2/3 -> Fourier2/1
  Fourier/1 -> To Workspace/1
  Demux2/1 -> Fourier/1
  In1/1 -> Demux2/1
  In2/1 -> Demux3/1

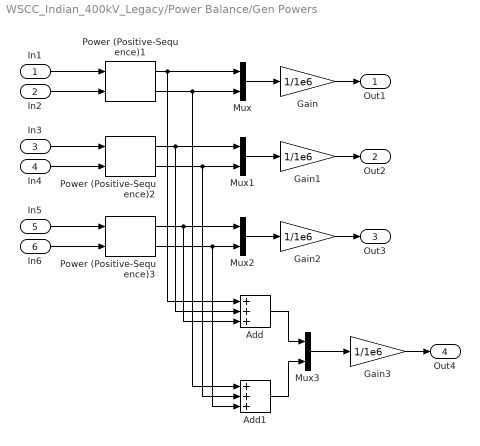
== system WSCC_Indian_400kV_Legacy/Power Balance/Gen Powers ==
  In1 : Inport
  In2 : Inport  Port=2
  In3 : Inport  Port=3
  In4 : Inport  Port=4
  In5 : Inport  Port=5
  In6 : Inport  Port=6
  Add : Sum  Inputs=+++
  Add1 : Sum  Inputs=+++
  Gain{,1..3} (4 alike) : Gain  Gain=1/1e6
  Mux{,1..3} (4 alike) : Mux  Inputs=2
  Power (Positive-Sequence)1 : spsPowerPositiveSequenceLib/Power (Positive-Sequence)  Freq=50  Vinit=[0, 0]  Iinit=[0, 0]  Ts=0
      settings: SourceProductBaseCode=PS
  Power (Positive-Sequence)2 : spsPowerPositiveSequenceLib/Power (Positive-Sequence)  Freq=50  Vinit=[0, 0]  Iinit=[0, 0]  Ts=0
      settings: SourceProductBaseCode=PS
  Power (Positive-Sequence)3 : spsPowerPositiveSequenceLib/Power (Positive-Sequence)  Freq=50  Vinit=[0, 0]  Iinit=[0, 0]  Ts=0
      settings: SourceProductBaseCode=PS
  Out1 : Outport  VectorParamsAs1DForOutWhenUnconnected=off
  Out2 : Outport  Port=2  VectorParamsAs1DForOutWhenUnconnected=off
  Out3 : Outport  Port=3  VectorParamsAs1DForOutWhenUnconnected=off
  Out4 : Outport  Port=4  VectorParamsAs1DForOutWhenUnconnected=off
  wires:
  Add/1 -> Mux3/1
  Mux3/1 -> Gain3/1
  Add1/1 -> Mux3/2
  Gain3/1 -> Out4/1
  Gain2/1 -> Out3/1
  Gain1/1 -> Out2/1
  Gain/1 -> Out1/1
  Mux2/1 -> Gain2/1
  Mux1/1 -> Gain1/1
  Mux/1 -> Gain/1
  Power (Positive-Sequence)3/2 -> Mux2/2, Add1/3
  Power (Positive-Sequence)3/1 -> Mux2/1, Add/3
  Power (Positive-Sequence)2/2 -> Mux1/2, Add1/2
  Power (Positive-Sequence)2/1 -> Mux1/1, Add/2
  Power (Positive-Sequence)1/2 -> Mux/2, Add1/1
  Power (Positive-Sequence)1/1 -> Mux/1, Add/1
  In6/1 -> Power (Positive-Sequence)3/2
  In5/1 -> Power (Positive-Sequence)3/1
  In4/1 -> Power (Positive-Sequence)2/2
  In3/1 -> Power (Positive-Sequence)2/1
  In2/1 -> Power (Positive-Sequence)1/2
  In1/1 -> Power (Positive-Sequence)1/1

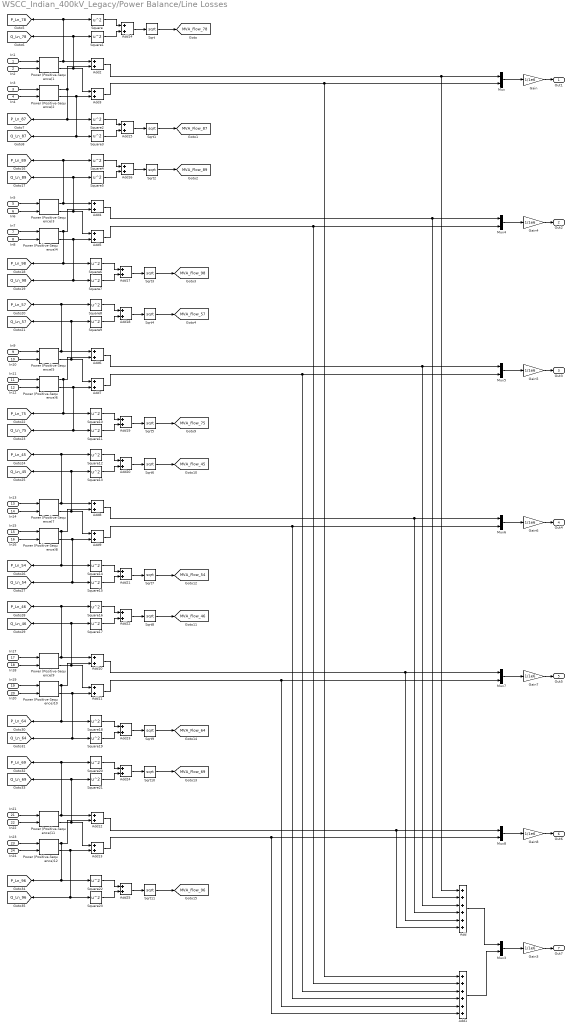
== system WSCC_Indian_400kV_Legacy/Power Balance/Line Losses ==
  In1 : Inport
  In2 : Inport  Port=2
  In3 : Inport  Port=3
  In4 : Inport  Port=4
  In5 : Inport  Port=5
  In6 : Inport  Port=6
  In7 : Inport  Port=7
  In8 : Inport  Port=8
  In9 : Inport  Port=9
  In10 : Inport  Port=10
  In11 : Inport  Port=11
  In12 : Inport  Port=12
  In13 : Inport  Port=13
  In14 : Inport  Port=14
  In15 : Inport  Port=15
  In16 : Inport  Port=16
  In17 : Inport  Port=17
  In18 : Inport  Port=18
  In19 : Inport  Port=19
  In20 : Inport  Port=20
  In21 : Inport  Port=21
  In22 : Inport  Port=22
  In23 : Inport  Port=23
  In24 : Inport  Port=24
  Add : Sum  Inputs=++++++
  Add1 : Sum  Inputs=++++++
  Add{2..25} (24 alike) : Sum
  Gain{,3..8} (7 alike) : Gain  Gain=1/1e6
  Mux{,3..8} (7 alike) : Mux  Inputs=2
  Power (Positive-Sequence){1..12} (12 alike) : spsPowerPositiveSequenceLib/Power (Positive-Sequence)  Freq=50  Vinit=[0, 0]  Iinit=[0, 0]  Ts=0
      settings: SourceProductBaseCode=PS
  Sqrt{,1..11} (12 alike) : Sqrt
  Square{,1..23} (24 alike) : Math  Operator=square  SignedPower=on
  Out1 : Outport  VectorParamsAs1DForOutWhenUnconnected=off
  Out2 : Outport  Port=2  VectorParamsAs1DForOutWhenUnconnected=off
  Out3 : Outport  Port=3  VectorParamsAs1DForOutWhenUnconnected=off
  Out4 : Outport  Port=4  VectorParamsAs1DForOutWhenUnconnected=off
  Out5 : Outport  Port=5  VectorParamsAs1DForOutWhenUnconnected=off
  Out6 : Outport  Port=6  VectorParamsAs1DForOutWhenUnconnected=off
  Out7 : Outport  Port=7  VectorParamsAs1DForOutWhenUnconnected=off
  tag scope: MVA_Flow_45=global, MVA_Flow_46=global, MVA_Flow_54=global, MVA_Flow_57=global, MVA_Flow_64=global, MVA_Flow_69=global, MVA_Flow_75=global, MVA_Flow_78=global, MVA_Flow_87=global, MVA_Flow_89=global, MVA_Flow_96=global, MVA_Flow_98=global, P_Ln_45=global, P_Ln_46=global, P_Ln_54=global, P_Ln_57=global, P_Ln_64=global, P_Ln_69=global, P_Ln_75=global, P_Ln_78=global, P_Ln_87=global, P_Ln_89=global, P_Ln_96=global, P_Ln_98=global, Q_Ln_45=global, Q_Ln_46=global, Q_Ln_54=global, Q_Ln_57=global, Q_Ln_64=global, Q_Ln_69=global, Q_Ln_75=global, Q_Ln_78=global, Q_Ln_87=global, Q_Ln_89=global, Q_Ln_96=global, Q_Ln_98=global
  wires:
  In1/1 -> Power (Positive-Sequence)1/1
  In2/1 -> Power (Positive-Sequence)1/2
  In3/1 -> Power (Positive-Sequence)2/1
  In4/1 -> Power (Positive-Sequence)2/2
  In5/1 -> Power (Positive-Sequence)3/1
  In6/1 -> Power (Positive-Sequence)3/2
  Mux/1 -> Gain/1
  Gain/1 -> Out1/1
  Gain3/1 -> Out7/1
  In12/1 -> Power (Positive-Sequence)6/2
  In11/1 -> Power (Positive-Sequence)6/1
  In10/1 -> Power (Positive-Sequence)5/2
  In9/1 -> Power (Positive-Sequence)5/1
  In8/1 -> Power (Positive-Sequence)4/2
  In7/1 -> Power (Positive-Sequence)4/1
  In19/1 -> Power (Positive-Sequence)10/1
  In20/1 -> Power (Positive-Sequence)10/2
  In21/1 -> Power (Positive-Sequence)11/1
  In22/1 -> Power (Positive-Sequence)11/2
  In23/1 -> Power (Positive-Sequence)12/1
  In24/1 -> Power (Positive-Sequence)12/2
  In18/1 -> Power (Positive-Sequence)9/2
  In17/1 -> Power (Positive-Sequence)9/1
  In16/1 -> Power (Positive-Sequence)8/2
  In15/1 -> Power (Positive-Sequence)8/1
  In14/1 -> Power (Positive-Sequence)7/2
  In13/1 -> Power (Positive-Sequence)7/1
  Power (Positive-Sequence)1/1 -> [P_Ln_78], Square/1, Add2/1
  Power (Positive-Sequence)1/2 -> [Q_Ln_78], Square1/1, Add3/1
  Add2/1 -> Mux/1, Add/1
  Add4/1 -> Mux4/1, Add/2
  Gain4/1 -> Out2/1
  Mux4/1 -> Gain4/1
  Mux5/1 -> Gain5/1
  Gain5/1 -> Out3/1
  Add6/1 -> Add/3, Mux5/1
  Add8/1 -> Mux6/1, Add/4
  Gain6/1 -> Out4/1
  Mux6/1 -> Gain6/1
  Mux7/1 -> Gain7/1
  Gain7/1 -> Out5/1
  Add10/1 -> Mux7/1, Add/5
  Add12/1 -> Mux8/1, Add/6
  Gain8/1 -> Out6/1
  Mux8/1 -> Gain8/1
  Add13/1 -> Add1/6, Mux8/2
  Add11/1 -> Add1/5, Mux7/2
  Add9/1 -> Add1/4, Mux6/2
  Add7/1 -> Add1/3, Mux5/2
  Add5/1 -> Add1/2, Mux4/2
  Add3/1 -> Add1/1, Mux/2
  Add/1 -> Mux3/1
  Add1/1 -> Mux3/2
  Mux3/1 -> Gain3/1
  Square/1 -> Add14/1
  Square1/1 -> Add14/2
  Add14/1 -> Sqrt/1
  Sqrt/1 -> [MVA_Flow_78]
  Sqrt1/1 -> [MVA_Flow_87]
  Add15/1 -> Sqrt1/1
  Square3/1 -> Add15/2
  Square2/1 -> Add15/1
  Power (Positive-Sequence)2/2 -> Square3/1, [Q_Ln_87], Add3/2
  Power (Positive-Sequence)2/1 -> [P_Ln_87], Square2/1, Add2/2
  Sqrt2/1 -> [MVA_Flow_89]
  Add16/1 -> Sqrt2/1
  Square5/1 -> Add16/2
  Square4/1 -> Add16/1
  Power (Positive-Sequence)3/2 -> [Q_Ln_89], Square5/1, Add5/1
  Power (Positive-Sequence)3/1 -> Square4/1, [P_Ln_89], Add4/1
  Power (Positive-Sequence)5/1 -> Square8/1, [P_Ln_57], Add6/1
  Power (Positive-Sequence)5/2 -> Square9/1, [Q_Ln_57], Add7/1
  Square8/1 -> Add18/1
  Square9/1 -> Add18/2
  Add18/1 -> Sqrt4/1
  Sqrt4/1 -> [MVA_Flow_57]
  Power (Positive-Sequence)4/1 -> Add4/2, Square6/1, [P_Ln_98]
  Power (Positive-Sequence)4/2 -> Add5/2, [Q_Ln_98], Square7/1
  Square6/1 -> Add17/1
  Square7/1 -> Add17/2
  Add17/1 -> Sqrt3/1
  Sqrt3/1 -> [MVA_Flow_98]
  Sqrt5/1 -> [MVA_Flow_75]
  Add19/1 -> Sqrt5/1
  Square11/1 -> Add19/2
  Square10/1 -> Add19/1
  Power (Positive-Sequence)6/2 -> Square11/1, [Q_Ln_75], Add7/2
  Power (Positive-Sequence)6/1 -> Square10/1, [P_Ln_75], Add6/2
  Sqrt6/1 -> [MVA_Flow_45]
  Add20/1 -> Sqrt6/1
  Square13/1 -> Add20/2
  Square12/1 -> Add20/1
  Power (Positive-Sequence)7/2 -> [Q_Ln_45], Square13/1, Add9/1
  Power (Positive-Sequence)7/1 -> Square12/1, [P_Ln_45], Add8/1
  Power (Positive-Sequence)9/1 -> [P_Ln_46], Square16/1, Add10/1
  Power (Positive-Sequence)9/2 -> [Q_Ln_46], Square17/1, Add11/1
  Square16/1 -> Add22/1
  Square17/1 -> Add22/2
  Add22/1 -> Sqrt8/1
  Sqrt8/1 -> [MVA_Flow_46]
  Power (Positive-Sequence)8/1 -> [P_Ln_54], Square14/1, Add8/2
  Power (Positive-Sequence)8/2 -> Square15/1, [Q_Ln_54], Add9/2
  Square14/1 -> Add21/1
  Square15/1 -> Add21/2
  Add21/1 -> Sqrt7/1
  Sqrt7/1 -> [MVA_Flow_54]
  Sqrt9/1 -> [MVA_Flow_64]
  Add23/1 -> Sqrt9/1
  Square19/1 -> Add23/2
  Square18/1 -> Add23/1
  Power (Positive-Sequence)10/2 -> Square19/1, [Q_Ln_64], Add11/2
  Power (Positive-Sequence)10/1 -> [P_Ln_64], Square18/1, Add10/2
  Sqrt10/1 -> [MVA_Flow_69]
  Add24/1 -> Sqrt10/1
  Square21/1 -> Add24/2
  Square20/1 -> Add24/1
  Power (Positive-Sequence)11/2 -> Square21/1, [Q_Ln_69], Add13/1
  Power (Positive-Sequence)11/1 -> Square20/1, [P_Ln_69], Add12/1
  Power (Positive-Sequence)12/1 -> Square22/1, [P_Ln_96], Add12/2
  Power (Positive-Sequence)12/2 -> Square23/1, [Q_Ln_96], Add13/2
  Square22/1 -> Add25/1
  Square23/1 -> Add25/2
  Add25/1 -> Sqrt11/1
  Sqrt11/1 -> [MVA_Flow_96]

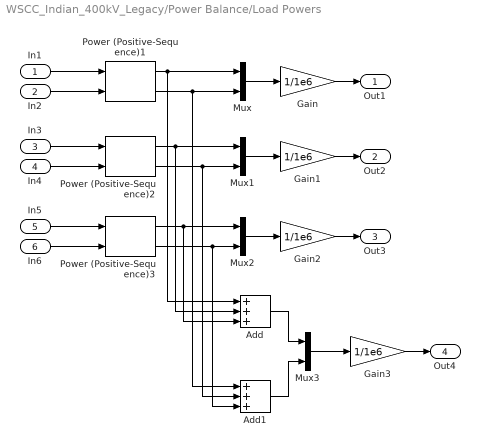
== system WSCC_Indian_400kV_Legacy/Power Balance/Load Powers ==
  In1 : Inport
  In2 : Inport  Port=2
  In3 : Inport  Port=3
  In4 : Inport  Port=4
  In5 : Inport  Port=5
  In6 : Inport  Port=6
  Add : Sum  Inputs=+++
  Add1 : Sum  Inputs=+++
  Gain{,1..3} (4 alike) : Gain  Gain=1/1e6
  Mux{,1..3} (4 alike) : Mux  Inputs=2
  Power (Positive-Sequence)1 : spsPowerPositiveSequenceLib/Power (Positive-Sequence)  Freq=50  Vinit=[0, 0]  Iinit=[0, 0]  Ts=0
      settings: SourceProductBaseCode=PS
  Power (Positive-Sequence)2 : spsPowerPositiveSequenceLib/Power (Positive-Sequence)  Freq=50  Vinit=[0, 0]  Iinit=[0, 0]  Ts=0
      settings: SourceProductBaseCode=PS
  Power (Positive-Sequence)3 : spsPowerPositiveSequenceLib/Power (Positive-Sequence)  Freq=50  Vinit=[0, 0]  Iinit=[0, 0]  Ts=0
      settings: SourceProductBaseCode=PS
  Out1 : Outport  VectorParamsAs1DForOutWhenUnconnected=off
  Out2 : Outport  Port=2  VectorParamsAs1DForOutWhenUnconnected=off
  Out3 : Outport  Port=3  VectorParamsAs1DForOutWhenUnconnected=off
  Out4 : Outport  Port=4  VectorParamsAs1DForOutWhenUnconnected=off
  wires:
  In1/1 -> Power (Positive-Sequence)1/1
  In2/1 -> Power (Positive-Sequence)1/2
  In3/1 -> Power (Positive-Sequence)2/1
  In4/1 -> Power (Positive-Sequence)2/2
  In5/1 -> Power (Positive-Sequence)3/1
  In6/1 -> Power (Positive-Sequence)3/2
  Power (Positive-Sequence)1/1 -> Add/1, Mux/1
  Power (Positive-Sequence)1/2 -> Add1/1, Mux/2
  Power (Positive-Sequence)2/1 -> Add/2, Mux1/1
  Power (Positive-Sequence)2/2 -> Add1/2, Mux1/2
  Power (Positive-Sequence)3/1 -> Add/3, Mux2/1
  Power (Positive-Sequence)3/2 -> Add1/3, Mux2/2
  Mux/1 -> Gain/1
  Mux1/1 -> Gain1/1
  Mux2/1 -> Gain2/1
  Gain/1 -> Out1/1
  Gain1/1 -> Out2/1
  Gain2/1 -> Out3/1
  Gain3/1 -> Out4/1
  Add1/1 -> Mux3/2
  Mux3/1 -> Gain3/1
  Add/1 -> Mux3/1

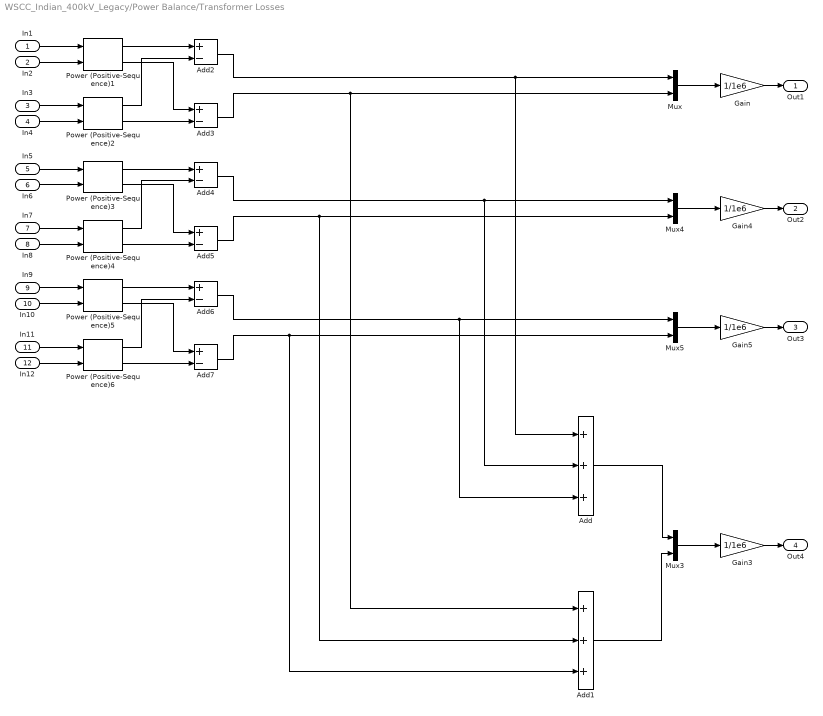
== system WSCC_Indian_400kV_Legacy/Power Balance/Transformer Losses ==
  In1 : Inport
  In2 : Inport  Port=2
  In3 : Inport  Port=3
  In4 : Inport  Port=4
  In5 : Inport  Port=5
  In6 : Inport  Port=6
  In7 : Inport  Port=7
  In8 : Inport  Port=8
  In9 : Inport  Port=9
  In10 : Inport  Port=10
  In11 : Inport  Port=11
  In12 : Inport  Port=12
  Add : Sum  Inputs=+++
  Add1 : Sum  Inputs=+++
  Add{2..7} (6 alike) : Sum  Inputs=+-
  Gain{,3..5} (4 alike) : Gain  Gain=1/1e6
  Mux{,3..5} (4 alike) : Mux  Inputs=2
  Power (Positive-Sequence){1..6} (6 alike) : spsPowerPositiveSequenceLib/Power (Positive-Sequence)  Freq=50  Vinit=[0, 0]  Iinit=[0, 0]  Ts=0
      settings: SourceProductBaseCode=PS
  Out1 : Outport  VectorParamsAs1DForOutWhenUnconnected=off
  Out2 : Outport  Port=2  VectorParamsAs1DForOutWhenUnconnected=off
  Out3 : Outport  Port=3  VectorParamsAs1DForOutWhenUnconnected=off
  Out4 : Outport  Port=4  VectorParamsAs1DForOutWhenUnconnected=off
  wires:
  Mux3/1 -> Gain3/1
  Add1/1 -> Mux3/2
  Add/1 -> Mux3/1
  Add3/1 -> Mux/2, Add1/1
  Add5/1 -> Mux4/2, Add1/2
  Add7/1 -> Mux5/2, Add1/3
  Add6/1 -> Mux5/1, Add/3
  Gain5/1 -> Out3/1
  Mux5/1 -> Gain5/1
  Mux4/1 -> Gain4/1
  Gain4/1 -> Out2/1
  Add4/1 -> Mux4/1, Add/2
  Add2/1 -> Mux/1, Add/1
  Power (Positive-Sequence)5/2 -> Add7/1
  Power (Positive-Sequence)6/2 -> Add7/2
  Power (Positive-Sequence)6/1 -> Add6/2
  Power (Positive-Sequence)5/1 -> Add6/1
  Power (Positive-Sequence)3/1 -> Add4/1
  Power (Positive-Sequence)4/1 -> Add4/2
  Power (Positive-Sequence)4/2 -> Add5/2
  Power (Positive-Sequence)3/2 -> Add5/1
  Power (Positive-Sequence)1/2 -> Add3/1
  Power (Positive-Sequence)2/2 -> Add3/2
  Power (Positive-Sequence)2/1 -> Add2/2
  Power (Positive-Sequence)1/1 -> Add2/1
  In7/1 -> Power (Positive-Sequence)4/1
  In8/1 -> Power (Positive-Sequence)4/2
  In9/1 -> Power (Positive-Sequence)5/1
  In10/1 -> Power (Positive-Sequence)5/2
  In11/1 -> Power (Positive-Sequence)6/1
  In12/1 -> Power (Positive-Sequence)6/2
  Gain3/1 -> Out4/1
  Gain/1 -> Out1/1
  Mux/1 -> Gain/1
  In6/1 -> Power (Positive-Sequence)3/2
  In5/1 -> Power (Positive-Sequence)3/1
  In4/1 -> Power (Positive-Sequence)2/2
  In3/1 -> Power (Positive-Sequence)2/1
  In2/1 -> Power (Positive-Sequence)1/2
  In1/1 -> Power (Positive-Sequence)1/1
